simulink model "Simulink_Lab1.1"  (R2026a)
settings: Solver=FixedStepDiscrete  StopTime=inf  FixedStep=0.001
undefined symbols (not defined in the file or in its folder): Blocking, Non
libraries: fl_lib x15, nesl_utility x15, ee_lib x5, amg_usbconverter_n_connect_lib x2
settings Model: Creator=pboon  LastModifiedBy=User

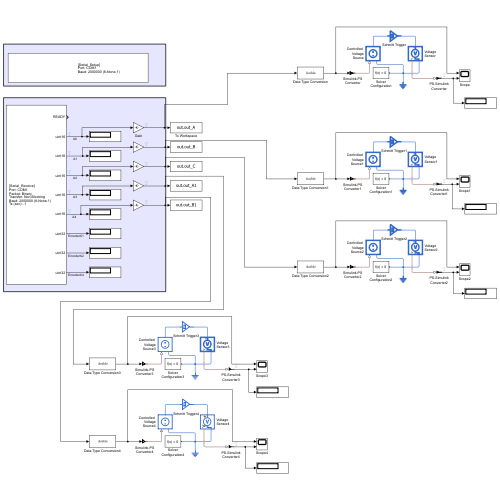
[thumbnail: Simulink's stored preview of the top-level diagram]
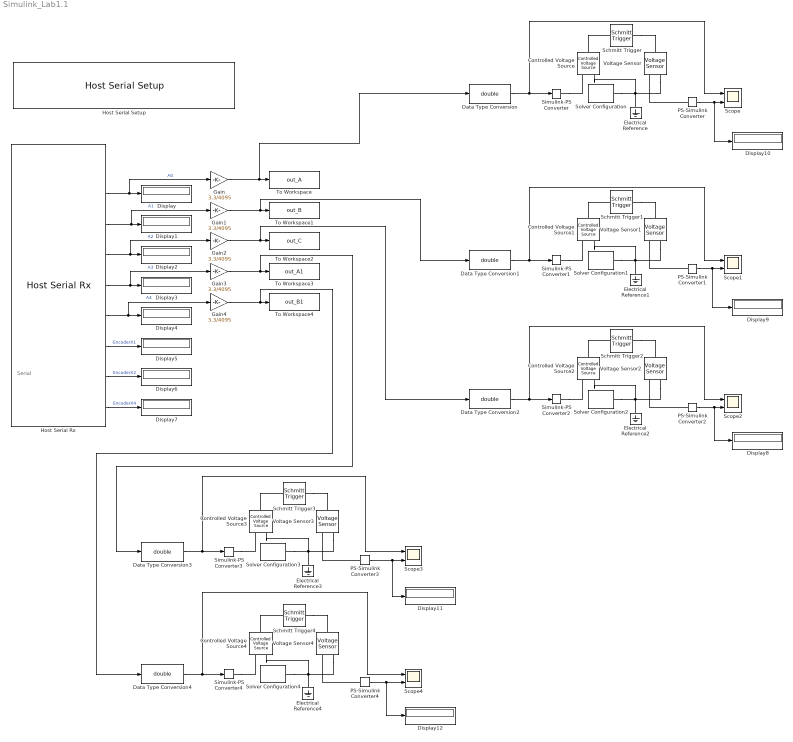
== system Simulink_Lab1.1 ==
  note: Serial
  Controlled Voltage Source{,1..4} (5 alike) : fl_lib/Electrical/Electrical Sources/Controlled Voltage Source
  Data Type Conversion{,1..4} (5 alike) : DataTypeConversion  OutDataTypeStr=double  SaturateOnIntegerOverflow=off  RndMeth=Floor
  Display{,1..12} (13 alike) : Display
  Electrical Reference{,1..4} (5 alike) : fl_lib/Electrical/Electrical Elements/Electrical Reference
  Gain{,1..4} (5 alike) : Gain  Gain=3.3/4095
  Host Serial Rx : amg_usbconverter_n_connect_lib/Host Serial Rx  conf=rx  port=<auto>  baudrate=2000000  databits=8  parity=None  stopbit=1  flowcontrol=None  transfer=Non-Blocking  timeout=5  packetmode=Binary  enableinitialvalues=off  initialvalues=[]  binheader='25'  binterminator='4E 4E'  porttype_double=0  porttype_single=0  porttype_int8=0  porttype_uint8=0  porttype_int16=0  porttype_uint16=5  porttype_int32=0  porttype_uint32=3  asciiformat='%d,%f'  rx_asciiterminator="CRLF (0x0D 0x0A - \"\\r\\n\")"  tx_asciiterminator="CRLF (0x0D 0x0A - \"\\r\\n\")"  sampletime=0.001  enablecustomportlabel=off  cinputportlabel=0  coutputportlabel=A  portpinstr=0  blockid=HostSerialRx  inputporttype=[]  inputportwidth=[]  inputportlabel={}  outputporttype=[3 5 5 5 5 5 7 7 7]  outputportwidth=[1 1 1 1 1 1 1 1 1]  outputportlabel={'READY','uint16','uint16','uint16','uint16','uint16','uint32','uint32','uint32'}  compat=0  optionstring=[]  autoport='COM1'
  Host Serial Setup : amg_usbconverter_n_connect_lib/Host Serial Setup  conf=setup  port=<auto>  baudrate=2000000  databits=8  parity=None  stopbit=1  flowcontrol=None  transfer=Blocking  timeout=2  packetmode=Binary  initialvalues=[]  binheader='7E 7E'  binterminator='03 03'  porttype_double=0  porttype_single=1  porttype_int8=0  porttype_uint8=0  porttype_int16=0  porttype_uint16=0  porttype_int32=0  porttype_uint32=2  asciiformat='%d %u %x'  rx_asciiterminator="CRLF (0x0D 0x0A - \"\\r\\n\")"  tx_asciiterminator="CRLF (0x0D 0x0A - \"\\r\\n\")"  sampletime=-1  enablecustomportlabel=off  cinputportlabel=0  coutputportlabel=A  portpinstr=0  blockid=HostSerialSetup  inputporttype=[]  inputportwidth=[]  inputportlabel={}  outputporttype=[]  outputportwidth=[]  outputportlabel={}  compat=0  optionstring=[]  autoport='COM1'
  PS-Simulink Converter{,1..4} (5 alike) : nesl_utility/PS-Simulink Converter  PhysicalDomain=network_engine_domain  SubClassName=ps_output  LeftPortType=input  RightPortType=output  PseudoPeriodic=off  Frequencies=[]  VectorFormat=inherit  Unit=inherit  AffineConversion=off
  Schmitt Trigger{,1..4} (5 alike) : ee_lib/Integrated Circuits/Logic/Schmitt Trigger  V_IL=1.0 V  V_IH=2.5 V  C_IN=5 pF  output_type=ee.enum.ic.outputType.linear  V_OL=0 V  V_OH=3.3 V  V_CC=5 V  V_meas=5 V  R_OUT=25 Ohm  R_OH=[25, 250] Ohm  I_OH=63 mA  R_OL=[30, 800] Ohm  I_OL=-45 mA  Delay=25 ns  Ron=5 Ohm  Vf=0.6 V  output_state=ee.enum.ic.initialState.low
  Scope{,1..4} (5 alike) : Scope  NumInputPorts=2
      Scope settings: ActiveDisplayYMinimum=-0.41249999999999987  ActiveDisplayYMaximum=3.7125
      Scope1 settings: ActiveDisplayYMinimum=-0.41249999999999987  ActiveDisplayYMaximum=3.7125
      Scope2 settings: ActiveDisplayYMinimum=-0.41249999999999987  ActiveDisplayYMaximum=3.7125  DataLoggingVariableName=ScopeData2
      Scope3 settings: ActiveDisplayYMinimum=-0.41249999999999987  ActiveDisplayYMaximum=3.7125  DataLoggingVariableName=ScopeData3
      Scope4 settings: ActiveDisplayYMinimum=-0.41249999999999987  ActiveDisplayYMaximum=3.7125  DataLoggingVariableName=ScopeData4
  Simulink-PS Converter{,1..4} (5 alike) : nesl_utility/Simulink-PS Converter  PhysicalDomain=network_engine_domain  SubClassName=ps_input  LeftPortType=input  RightPortType=output  PseudoPeriodic=off  Frequencies=[]  NoiseDistribution=none  NoiseParameters=[]  Unit=1  AffineConversion=off  FilteringAndDerivatives=provide  SimscapeFilterOrder=1  InputFilterTimeConstant=0.001  UdotUserProvided=0
  Solver Configuration{,1..4} (5 alike) : nesl_utility/Solver Configuration  PhysicalDomain=network_engine_domain  SubClassName=solver  LeftPortType=input  RightPortType=generic  Tones=[]  Harmonics=[]  SimulateNoise=off  Profile=off  UseLocalSampling=off  EnableSwitchedLinearOptims=on  FrequencyDomain=off  UseCCode=off  RelTol=0.001  AbsTol=0.001  MinStep=1e-09  ToWorkspace=off  RevertToSquareIcSolve=off  NumHomotopyIterations=100  PhasorMode=off  PhasorModeNumHarmonics=1  ConsistencySolver=NEWTON_XTOL_AFTER_FTOL  CanonicalOrdering=CANONICAL  OptimizeIntermediates=OPTIMIZED  IndexReductionMethod=DerivativeReplacement  DoDC=off  ResidualTolerance=1e-09  ConsistencyTolSource=GLOBAL  ConsistencyAbsTol=0.001  ConsistencyRelTol=0.001  ConsistencyTolFactor=0.001  UseLocalSolver=on  LocalSolverChoice=NE_BACKWARD_EULER_ADVANCER  ResolveIndetEquations=on  FunctionEvalNumThread=1  LocalSolverSampleTime=0.001  DoFixedCost=off  MaxNonlinIter=3  MaxModeIter=2  ComputeImpulses=off  ImpulseIterations=2  LinearAlgebra=auto  LinearAlgebraNumThread=0  EquationFormulation=NE_TIME_EF  DelaysMemoryBudget=1024  AutomaticFiltering=on  FilteringTimeConstant=0.001  PartitionStorageMethod=AS_NEEDED  PartitionMemoryBudget=1024  PartitionMethod=ROBUST  MultibodyUseLocalSolver=off  MultibodyLocalSolverChoice=ODE1  MultibodyLocalSolverSampleTime=0.001
  To Workspace : ToWorkspace  VariableName=out_A  SaveFormat=Timeseries  SampleTime=-1
  To Workspace1 : ToWorkspace  VariableName=out_B  SaveFormat=Timeseries  SampleTime=-1
  To Workspace2 : ToWorkspace  VariableName=out_C  SaveFormat=Timeseries  SampleTime=-1
  To Workspace3 : ToWorkspace  VariableName=out_A1  SaveFormat=Timeseries  SampleTime=-1
  To Workspace4 : ToWorkspace  VariableName=out_B1  SaveFormat=Timeseries  SampleTime=-1
  Voltage Sensor{,1..4} (5 alike) : fl_lib/Electrical/Electrical Sensors/Voltage Sensor
  wires:
  Host Serial Rx/2 -> Gain/1, Display/1  "A0"
  Host Serial Rx/3 -> Gain1/1, Display1/1  "A1"
  Host Serial Rx/4 -> Gain2/1, Display2/1  "A2"
  Host Serial Rx/5 -> Gain3/1, Display3/1  "A3"
  Host Serial Rx/6 -> Gain4/1, Display4/1  "A4"
  Host Serial Rx/7 -> Display5/1  "EncoderX1"
  Host Serial Rx/8 -> Display6/1  "EncoderX2"
  Host Serial Rx/9 -> Display7/1  "EncoderX4"
  Gain/1 -> Data Type Conversion/1, To Workspace/1
  Gain1/1 -> Data Type Conversion1/1, To Workspace1/1
  Gain2/1 -> Data Type Conversion2/1, To Workspace2/1
  Gain3/1 -> Data Type Conversion3/1, To Workspace3/1
  Gain4/1 -> Data Type Conversion4/1, To Workspace4/1
  PS-Simulink Converter/1 -> Display10/1, Scope/2
  Data Type Conversion/1 -> Scope/1, Simulink-PS Converter/1
  Data Type Conversion1/1 -> Scope1/1, Simulink-PS Converter1/1
  PS-Simulink Converter1/1 -> Display9/1, Scope1/2
  Data Type Conversion2/1 -> Scope2/1, Simulink-PS Converter2/1
  PS-Simulink Converter2/1 -> Display8/1, Scope2/2
  PS-Simulink Converter3/1 -> Display11/1, Scope3/2
  Data Type Conversion3/1 -> Scope3/1, Simulink-PS Converter3/1
  PS-Simulink Converter4/1 -> Display12/1, Scope4/2
  Data Type Conversion4/1 -> Scope4/1, Simulink-PS Converter4/1
  connections:
  Controlled Voltage Source/LConn1 -- Schmitt Trigger/LConn1
  Schmitt Trigger/RConn1 -- Voltage Sensor/LConn1
  Solver Configuration/RConn1 -- Controlled Voltage Source/RConn2 -- Voltage Sensor/RConn2 -- Electrical Reference/LConn1
  PS-Simulink Converter/LConn1 -- Voltage Sensor/RConn1
  Simulink-PS Converter/RConn1 -- Controlled Voltage Source/RConn1
  Solver Configuration1/RConn1 -- Electrical Reference1/LConn1 -- Controlled Voltage Source1/RConn2 -- Voltage Sensor1/RConn2
  PS-Simulink Converter1/LConn1 -- Voltage Sensor1/RConn1
  Schmitt Trigger1/RConn1 -- Voltage Sensor1/LConn1
  Simulink-PS Converter1/RConn1 -- Controlled Voltage Source1/RConn1
  Controlled Voltage Source1/LConn1 -- Schmitt Trigger1/LConn1
  Solver Configuration2/RConn1 -- Electrical Reference2/LConn1 -- Controlled Voltage Source2/RConn2 -- Voltage Sensor2/RConn2
  PS-Simulink Converter2/LConn1 -- Voltage Sensor2/RConn1
  Schmitt Trigger2/RConn1 -- Voltage Sensor2/LConn1
  Simulink-PS Converter2/RConn1 -- Controlled Voltage Source2/RConn1
  Controlled Voltage Source2/LConn1 -- Schmitt Trigger2/LConn1
  Solver Configuration3/RConn1 -- Electrical Reference3/LConn1 -- Controlled Voltage Source3/RConn2 -- Voltage Sensor3/RConn2
  Schmitt Trigger3/RConn1 -- Voltage Sensor3/LConn1
  PS-Simulink Converter3/LConn1 -- Voltage Sensor3/RConn1
  Controlled Voltage Source3/LConn1 -- Schmitt Trigger3/LConn1
  Simulink-PS Converter3/RConn1 -- Controlled Voltage Source3/RConn1
  Solver Configuration4/RConn1 -- Electrical Reference4/LConn1 -- Controlled Voltage Source4/RConn2 -- Voltage Sensor4/RConn2
  Schmitt Trigger4/RConn1 -- Voltage Sensor4/LConn1
  PS-Simulink Converter4/LConn1 -- Voltage Sensor4/RConn1
  Controlled Voltage Source4/LConn1 -- Schmitt Trigger4/LConn1
  Simulink-PS Converter4/RConn1 -- Controlled Voltage Source4/RConn1
